simulink model "lqr_110"  (Simulink 8.5)
settings: Solver=ode45  StartTime=0.0  StopTime=10.0  RelTol=1e-3
values from neighbouring files (symbols this model uses):
  AMin = [ ... (first row only)    [LqrObs.m]    (also in LqrObs1_15.m)
  Aoss = AMin-L*ClocalMin    [LqrObs.m]    (also in LqrObs1_15.m)
  BMin = [ ... (first row only)    [LqrObs.m]    (also in LqrObs1_15.m)
  Boss = [BMin-L*D L]    [LqrObs.m]    (also in LqrObs1_15.m)
  ClocalMin = [ ... (first row only)    [LqrObs.m]    (also in LqrObs1_15.m)
  Coss = eye(size(AMin))    [LqrObs.m]    (also in LqrObs1_15.m)
  D = zeros(4,4)    [LqrObs.m]    (also in LqrObs1_15.m)
  Doss = zeros(size(Boss))    [LqrObs.m]    (also in LqrObs1_15.m)
  K = lqr(AMin,BMin,Qie,Rie)    [LqrObs.m]    (also in LqrObs1_15.m)
  L = place(AMin',ClocalMin',P)'    [LqrObs.m]    (also in LqrObs1_15.m)
  refs = [10 0 0 0 45 0 0 0 ]    [LqrObs.m]    (also in LqrObs1_15.m)
libraries: simulink_extras x2
settings Model: Creator=UserK  LastModifiedBy=UserK
settings DataIOCC: SignalLoggingSaveFormat=Dataset
settings OptimizationCC: ExpressionDepthLimit=128
settings DebuggingCC: UnderspecifiedInitializationDetection=Simplified  MergeDetectMultiDrivingBlocksExec=error  FcnCallInpInsideContextMsg=EnableAllAsError  StateNameClashWarn=none
settings GRTTargetCC: CombineOutputUpdateFcns=on  GRTInterface=off

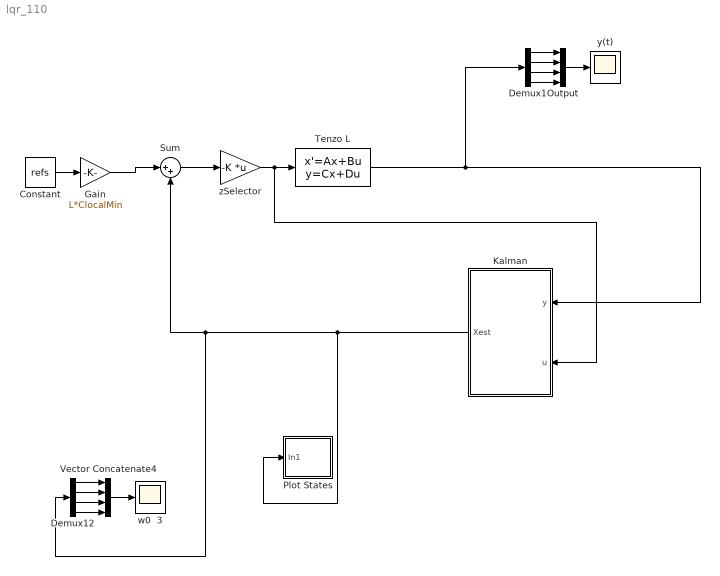
== system lqr_110 ==
  Constant : Constant  Value=refs
  Demux1 : Demux
  Demux12 : Demux
  Gain : Gain  Gain=L*ClocalMin
  Kalman : Subsystem
  Output : Concatenate  NumInputs=4
  Plot States : Subsystem
  Sum : Sum  Inputs=|++
  Tenzo L : StateSpace  A=AMin  B=BMin  C=ClocalMin  D=D  X0=[10 0 10 0 180 0 0 0 ]
  Vector Concatenate4 : Concatenate  NumInputs=4
  w0  3 : Scope
      settings: YMin=2500  YMax=7000  SaveName=ScopeData36
  y(t) : Scope
      settings: YMin=2500  YMax=7000  SaveName=ScopeData20
  zSelector : Gain  Gain=-K  Multiplication=Matrix(K*u)
  wires:
  Tenzo L/1 -> Demux1/1, Kalman/1(y)
  Kalman/1(Xest) -> Plot States/1(In1), Sum/2, Demux12/1
  Demux12/1 -> Vector Concatenate4/1
  Demux12/2 -> Vector Concatenate4/2
  Demux12/3 -> Vector Concatenate4/3
  Demux12/4 -> Vector Concatenate4/4
  Vector Concatenate4/1 -> w0  3/1
  Demux1/1 -> Output/1
  Demux1/2 -> Output/2
  Demux1/3 -> Output/3
  Demux1/4 -> Output/4
  Output/1 -> y(t)/1
  Constant/1 -> Gain/1
  Gain/1 -> Sum/1
  Sum/1 -> zSelector/1
  zSelector/1 -> Kalman/2(u), Tenzo L/1

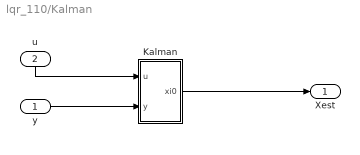
== system lqr_110/Kalman ==
  y : Inport
  u : Inport  Port=2
  Kalman : Subsystem
  Xest : Outport
  wires:
  Kalman/1(xi0) -> Xest/1
  u/1 -> Kalman/1(u)
  y/1 -> Kalman/2(y)

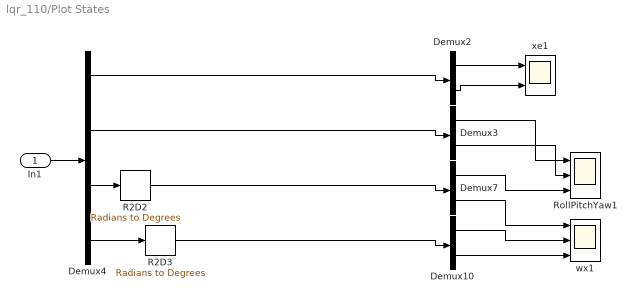
== system lqr_110/Plot States ==
  In1 : Inport
  Demux{2..3,7,10} (4 alike) : Demux  Outputs=2
  Demux4 : Demux
  R2D2 : simulink_extras/Transformations/Radians to Degrees
  R2D3 : simulink_extras/Transformations/Radians to Degrees
  RollPitchYaw1 : Scope  NumInputPorts=3
      settings: YMin=-5~-5~-5  YMax=5~5~5  SaveName=ScopeData21
  wx1 : Scope  NumInputPorts=3
      settings: TimeRange=15  YMin=-5~-5~-5  YMax=5~5~5  SaveName=ScopeData24
  xe1 : Scope  NumInputPorts=2
      settings: TimeRange=3  YMin=1.6e-05~1.6e-05  YMax=3e-05~3e-05  SaveName=ScopeData25
  wires:
  Demux4/1 -> Demux2/1
  Demux4/2 -> Demux3/1
  Demux4/4 -> R2D3/1
  Demux2/1 -> xe1/1
  Demux2/2 -> xe1/2
  R2D2/1 -> Demux7/1
  R2D3/1 -> Demux10/1
  Demux4/3 -> R2D2/1
  In1/1 -> Demux4/1
  Demux10/2 -> wx1/3
  Demux10/1 -> wx1/2
  Demux7/2 -> wx1/1
  Demux7/1 -> RollPitchYaw1/3
  Demux3/2 -> RollPitchYaw1/2
  Demux3/1 -> RollPitchYaw1/1

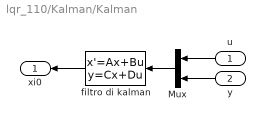
== system lqr_110/Kalman/Kalman ==
  u : Inport
  y : Inport  Port=2
  Mux : Mux  Inputs=[4 4]
  filtro di kalman : StateSpace  A=Aoss  B=Boss  C=Coss  D=Doss  X0=[0 0 0 0 0 0 0 0]
  xi0 : Outport
  wires:
  Mux/1 -> filtro di kalman/1
  u/1 -> Mux/1
  filtro di kalman/1 -> xi0/1
  y/1 -> Mux/2
